simulink model "Test_Logic_Operation_Bitwise_AND"  (Simulink 8.1)
settings: Solver=VariableStepDiscrete  StartTime=0.0  StopTime=len  RelTol=1e-3
libraries: Logic_Operations_Lib x1
settings Model: Creator=uzivatel  LastModifiedBy=uzivatel
settings DataIOCC: SignalLoggingSaveFormat=Dataset
settings OptimizationCC: ExpressionDepthLimit=128
settings DebuggingCC: FcnCallInpInsideContextMsg=EnableAllAsError
settings GRTTargetCC: CombineOutputUpdateFcns=on  GRTInterface=off

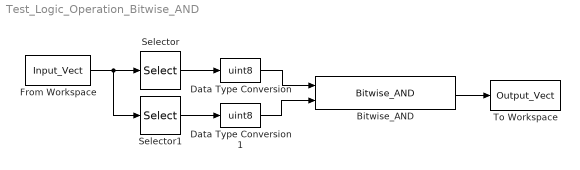
== system Test_Logic_Operation_Bitwise_AND ==
  Bitwise_AND : Logic_Operations_Lib/Logic_Operations_Lib/Bitwise_AND
  Data Type Conversion : DataTypeConversion  OutDataTypeStr=uint8
  Data Type Conversion1 : DataTypeConversion  OutDataTypeStr=uint8
  From Workspace : FromWorkspace  VariableName=Input_Vect  SampleTime=1  Interpolate=off  OutputAfterFinalValue=Holding final value
  Selector : Selector  IndexMode=Zero-based  InputPortWidth=2  SampleTime=1  IndexOptions=Index vector (dialog)  Indices=0  OutputSizes=1
  Selector1 : Selector  IndexMode=Zero-based  InputPortWidth=2  SampleTime=1  IndexOptions=Index vector (dialog)  Indices=1  OutputSizes=1
  To Workspace : ToWorkspace  VariableName=Output_Vect  SampleTime=1
  wires:
  Data Type Conversion1/1 -> Bitwise_AND/2
  Data Type Conversion/1 -> Bitwise_AND/1
  From Workspace/1 -> Selector1/1, Selector/1
  Bitwise_AND/1 -> To Workspace/1
  Selector/1 -> Data Type Conversion/1
  Selector1/1 -> Data Type Conversion1/1
